simulink model "readValuesCl"  (R2022a)
settings: Solver=VariableStepAuto  StartTime=0.0  StopTime=10.0  RelTol=1e-3
values from neighbouring files (symbols this model uses):
  Ki = 0    [initcl.m]
  Kp = 0    [initcl.m]
  SetpointCl = 0    [initcl.m]
settings Model: Creator=Usuario  LastModifiedBy=Usuario
settings DebuggingCC: AlgebraicLoopMsg=none

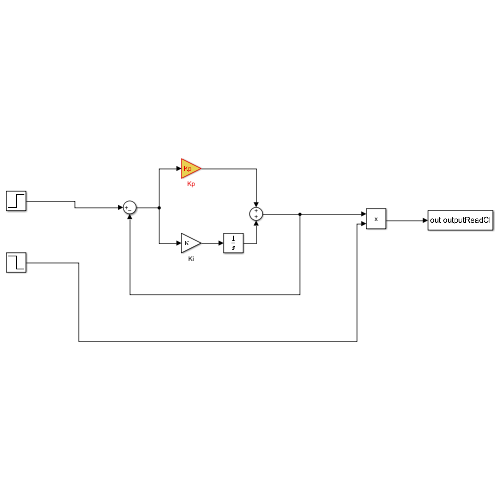
[thumbnail: Simulink's stored preview of the top-level diagram]
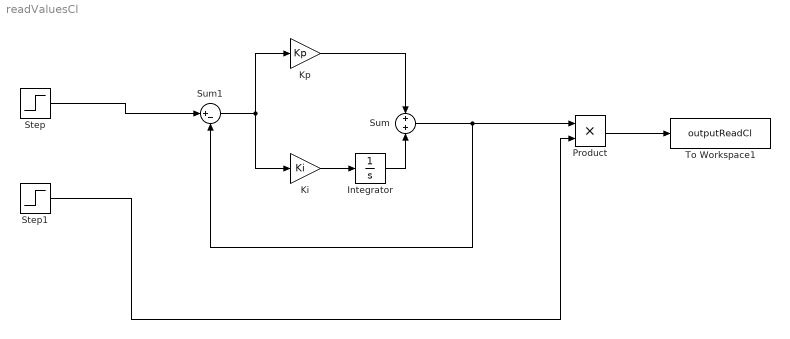
== system readValuesCl ==
  Integrator : Integrator
  Ki : Gain  Gain=Ki
  Kp : Gain  Gain=Kp
  Product : Product
  Step : Step  After=SetpointCl  SampleTime=0
  Step1 : Step  Time=9  Before=1  After=0  SampleTime=0
  Sum : Sum
  Sum1 : Sum  Inputs=|+-
  To Workspace1 : ToWorkspace  VariableName=outputReadCl  SampleTime=-1
  wires:
  Sum1/1 -> Kp/1, Ki/1
  Ki/1 -> Integrator/1
  Kp/1 -> Sum/1
  Integrator/1 -> Sum/2
  Sum/1 -> Product/1, Sum1/2
  Step/1 -> Sum1/1
  Step1/1 -> Product/2
  Product/1 -> To Workspace1/1
